simulink model "linmodel_eq1_discr2_lqr"  (R2019a)
settings: Solver=VariableStepAuto  StartTime=0.0  StopTime=30  RelTol=1e-3
InitFcn:
  | lin_discr_model
values from neighbouring files (symbols this model uses):
  A_eq1_d = sysd1.A    [lin_discr_model_tryouts.m]
  B_eq1_d = sysd1.B    [lin_discr_model_tryouts.m]
  C_eq1_d = sysd1.C    [lin_discr_model_tryouts.m]
  Ts = 0.01    [lin_discr_model_tryouts.m]
undefined symbols (not defined in the file or in its folder): K1, L2
settings Model: Creator=jessi  LastModifiedBy=jessi

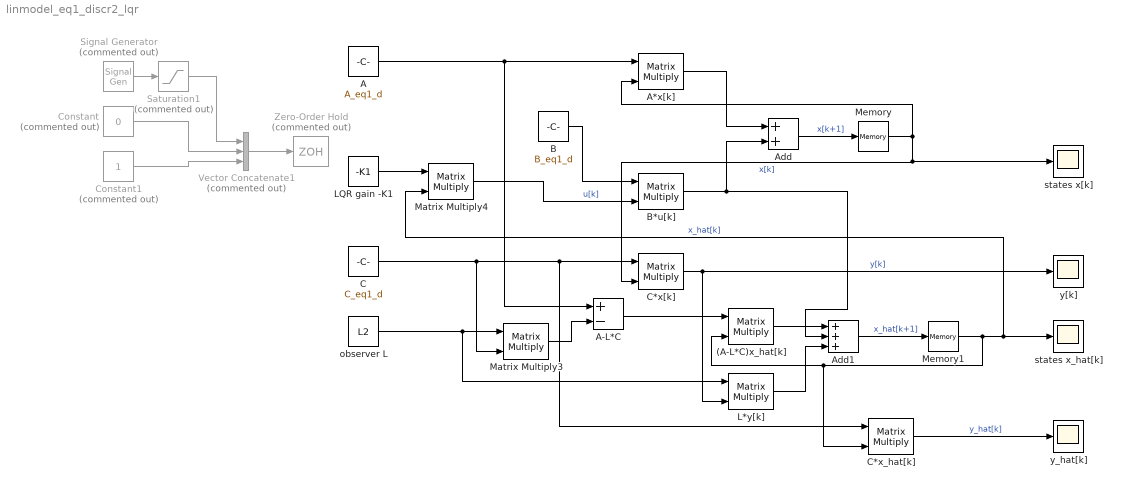
== system linmodel_eq1_discr2_lqr ==
  (A-L*C)x_hat[k] : Product  Multiplication=Matrix(*)
  A : Constant  Value=A_eq1_d  SampleTime=Ts
  A*x[k] : Product  Multiplication=Matrix(*)
  A-L*C : Sum  Inputs=+-
  Add : Sum
  Add1 : Sum  Inputs=+++
  B : Constant  Value=B_eq1_d  SampleTime=Ts
  B*u[k] : Product  Multiplication=Matrix(*)
  C : Constant  Value=C_eq1_d  SampleTime=Ts
  C*x[k] : Product  Multiplication=Matrix(*)
  C*x_hat[k] : Product  Multiplication=Matrix(*)
  Constant : Constant  Commented=on  Value=0
  Constant1 : Constant  Commented=on
  L*y[k] : Product  Multiplication=Matrix(*)
  LQR gain -K1 : Constant  Value=-K1
  Matrix Multiply3 : Product  Multiplication=Matrix(*)
  Matrix Multiply4 : Product  Multiplication=Matrix(*)
  Memory : Memory  InitialCondition=[pi;0;0;0]
  Memory1 : Memory  InitialCondition=[pi;0;0;0]
  Saturation1 : Saturate  Commented=on  UpperLimit=1  LowerLimit=-1
  Signal Generator : SignalGenerator  Commented=on  WaveForm=square  Amplitude=-0.3
  Vector Concatenate1 : Concatenate  Commented=on  NumInputs=3
  Zero-Order Hold : ZeroOrderHold  Commented=on  SampleTime=Ts
  observer L : Constant  Value=L2  SampleTime=Ts
  states x[k] : Scope
  states x_hat[k] : Scope
  y[k] : Scope
  y_hat[k] : Scope
  wires:
  Constant/1 -> Vector Concatenate1/2
  Signal Generator/1 -> Saturation1/1
  Saturation1/1 -> Vector Concatenate1/1
  Constant1/1 -> Vector Concatenate1/3
  Vector Concatenate1/1 -> Zero-Order Hold/1
  B/1 -> B*u[k]/1
  A/1 -> A-L*C/1, A*x[k]/1
  A*x[k]/1 -> Add/1
  B*u[k]/1 -> Add1/2, Add/2
  Add/1 -> Memory/1  "x[k+1]"
  Memory/1 -> A*x[k]/2, states x[k]/1, C*x[k]/2  "x[k]"
  C/1 -> Matrix Multiply3/2, C*x_hat[k]/1, C*x[k]/1
  C*x[k]/1 -> L*y[k]/2, y[k]/1  "y[k]"
  observer L/1 -> L*y[k]/1, Matrix Multiply3/1
  Matrix Multiply3/1 -> A-L*C/2
  A-L*C/1 -> (A-L*C)x_hat[k]/1
  (A-L*C)x_hat[k]/1 -> Add1/1
  L*y[k]/1 -> Add1/3
  Add1/1 -> Memory1/1  "x_hat[k+1]"
  Memory1/1 -> Matrix Multiply4/2, states x_hat[k]/1, C*x_hat[k]/2, (A-L*C)x_hat[k]/2  "x_hat[k]"
  C*x_hat[k]/1 -> y_hat[k]/1  "y_hat[k]"
  LQR gain -K1/1 -> Matrix Multiply4/1
  Matrix Multiply4/1 -> B*u[k]/2  "u[k]"
